simulink model "sgMdl_CAN_J1939Loopback"  (R2024b)
settings: Solver=FixedStepAuto  StartTime=0.0  StopTime=inf  RelTol=1e-3  EnableMultiTasking=on
undefined symbols (not defined in the file): Down, ET1_EMS, IO602, Pull, TCFG2_TECU
libraries: j1939protocollib x8, speedgoatlib_IO602_4 x5, simulink x3, slrtj1939tllib x2
Description:
  | CAN - Working with J1939
settings Model: ModifiedByFormat=Speedgoat  SimulationMode=external  ExtModeEnableFloating=off  ExtModeTrigDuration=100000  VariantFading=off  Creator=Speedgoat  LastModifiedBy=Speedgoat
settings SolverCC: ConcurrentTasks=on  AlgebraicLoopSolver=TrustRegion  PositivePriorityOrder=on  AutoInsertRateTranBlk=on  InsertRTBMode=Never (minimum delay)
settings DataIOCC: SaveFormat=StructureWithTime
settings OptimizationCC: BlockReduction=off  OptimizeBlockIOStorage=off  BufferReuse=off  GlobalBufferReuse=off  ExpressionFolding=off  LocalBlockOutputs=off  OptimizeDataStoreBuffers=off  BusAssignmentInplaceUpdate=off
settings DebuggingCC: InheritedTsInSrcMsg=none  TasksWithSamePriorityMsg=none  ParameterPrecisionLossMsg=none  UnconnectedInputMsg=warning  UnconnectedOutputMsg=warning  UnconnectedLineMsg=warning
settings HardwareCC: ProdBitPerLong=64  ProdLongLongMode=on  ProdHWDeviceType=Intel->x86-64 (Linux 64)
settings ModelReferenceCC: EnableRefExpFcnMdlSchedulingChecks=on
settings SFSimCC: CustomCodeUndefinedFunction=UseInterfaceOnly
settings RTWCC: Description=Speedgoat Real-Time Target Machine  SystemTargetFile=speedgoat.tlc  TemplateMakefile=slrealtime_default_tmf  Toolchain=Simulink Real-Time Toolchain  BuildConfiguration=Faster Runs  TargetLang=C++  GPUComputeCapability=3.5  DLArmComputeVersion=19.05
settings SimulinkRealTimeTargetCC: SubcomponentCodeInterfacePackaging=Reusable function  InstructionSetFMA=off  LogToMDFFile=off  SLRTFileLogMaxRuns=10  UseGCCFastMath=on
settings ConfigComp: CovBoundaryAbsTol=1.0e-5

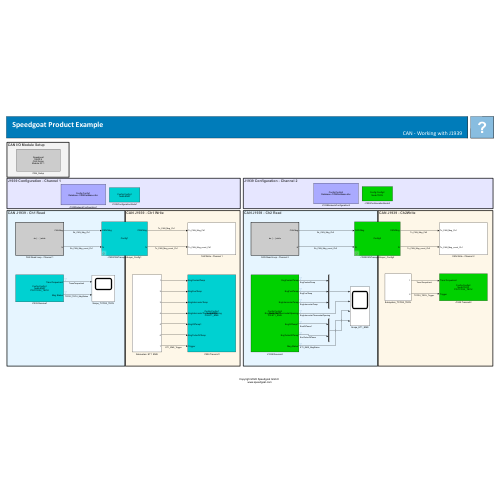
[thumbnail: Simulink's stored preview of the top-level diagram]
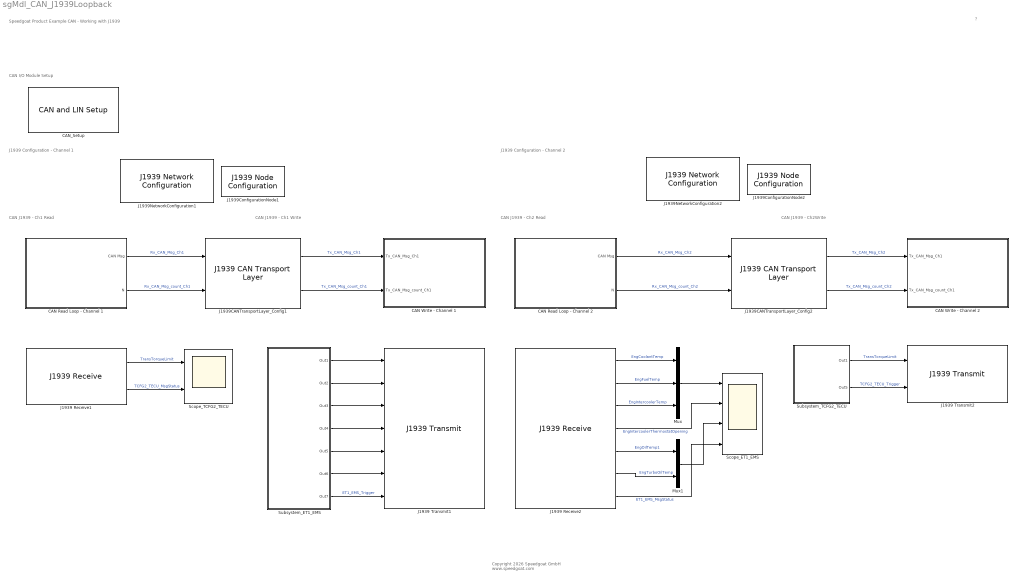
== system sgMdl_CAN_J1939Loopback ==
  note: CAN I/O Module Setup
  note: J1939 Configuration - Channel 1
  note: CAN J1939 - Ch2 Read
  note: CAN J1939 - Ch2Write
  note: CAN J1939 - Ch1 Read
  note: CAN J1939 - Ch1 Write
  note: J1939 Configuration - Channel 2
  note: Speedgoat Product Example
      | CAN - Working with J1939
  note: ?
  note: Copyright 2026 Speedgoat GmbH
      |  www.speedgoat.com
  CAN Read Loop - Channel 1 : Subsystem  TreatAsAtomicUnit=on
  CAN Read Loop - Channel 2 : Subsystem  TreatAsAtomicUnit=on
  CAN Write - Channel 1 : Subsystem
  CAN Write - Channel 2 : Subsystem
  CAN_Setup : speedgoatlib_IO602_4/CAN and LIN Setup   moduleInitValues="[6022     1     1    -1    -1]"  id=1  moduleType=IO602-2  pciSlot=-1  canChn1=CAN (HS)  canChn2=CAN (HS)  canChn3=Disabled  canChn4=Disabled  linChn1=Disabled  linChn2=Disabled  canInitStructArray=[]  canTermStructArray=[]  gpioChnx=Disabled  canChn1InitValues="[2   2   8   1  16   3  19   2   2   5   2   0]"  arbBdrChn1=500 kBaud  clockDividerChn1=Enable  arbManBdrChn1=[8,1,16,3]  fdBdrChn1=5.0 MBaud  fdManBdrChn1=[2,2,5,2]  termResistor1=off  canChn2InitValues="[2   2   8   1  16   3  19   2   2   5   2   0]"  arbBdrChn2=500 kBaud  clockDividerChn2=Enable  arbManBdrChn2=[8,1,16,3]  fdBdrChn2=5.0 MBaud  fdManBdrChn2=[2,2,5,2]  termResistor2=off  canChn3InitValues="[1   0   2   8  31   8  19   2   2   5   2   0]"  arbBdrChn3=1.0 MBaud  clockDividerChn3=Enable  arbManBdrChn3=[2,8,31,8]  fdBdrChn3=5.0 MBaud  fdManBdrChn3=[2,2,5,2]  termResistor3=off  canChn4InitValues="[1   0   2   8  31   8  19   2   2   5   2   0]"  arbBdrChn4=1.0 MBaud  clockDividerChn4=Enable  arbManBdrChn4=[2,8,31,8]  fdBdrChn4=5.0 MBaud  fdManBdrChn4=[2,2,5,2]  termResistor4=off  linChn1InitValues="[0  9600]"  linBtrChn1=9600  linChn2InitValues="[0  9600]"  linBtrChn2=9600  doInitTermStruct="[0  5  0  0  0]"  parDoChannels=[1 2]  parDoVoltage=5  parDoInitValues=0  parDoReset=1  parNumOfDoS=0  parDiChannels=[3 4]  parDiVoltage=5  parDiPull=Pull-Down
      settings: SourceProductName=Simulink Real-Time: Speedgoat I/O Blockset
  J1939 Receive1 : j1939protocollib/J1939 Receive  Priority=-1  ConfigName=Config1  NodeName=EMS  PGList=TCFG2_TECU(65099)  PGName=TCFG2_TECU  MsgLength=8  SignalInfo=TransTorqueLimit$0$16$1$2$1$0$1$0$0$64255$Nm$1845$#  NSignals=1  StartBits=str2num('[double(0)]')  SignalSizes=str2num('[double(16)]')  ByteOrders=str2num('[int32(1)]')  DataTypes=str2num('[int32(2)]')  MultiplexTypes=str2num('[int32(1)]')  MultiplexValues=str2num('[double(0)]')  Factors=str2num('[double(1)]')  Offsets=str2num('[double(0)]')  Minimums=str2num('[double(0)]')  Maximums=str2num('[double(64255)]')  Units=0  SPN=str2num('[double(1845)]')  Comment=0  SrcAddrFilter=Allow all  SrcAddress=255  DestAddrFilter=1  outputNew=on  SampleTime=0.01  ApplyMinMax=off
  J1939 Receive2 : j1939protocollib/J1939 Receive  Priority=-1  ConfigName=Config2  NodeName=TECU  PGList=ET1_EMS(65262)  PGName=ET1_EMS  MsgLength=8  SignalInfo=EngCoolantTemp$0$8$1$2$1$0$1$-40$-40$210$deg$110$#EngFuelTemp$8$8$1$2$1$0$1$-40$-40$210$deg$174$#EngIntercoolerTemp$48$8$1$2$1$0$1$-40$-40$210$deg$52$#EngIntercoolerThermostatOpening$56$8$1$2$1$0$4.000000e-01$0$0$100$%$1134$#EngOilTemp1$16$16$1$2$1$0$3.125000e-02$-273$-273$1735$deg$175$#EngTurboOilTemp$32$16$1$2$1$0$3.125000e-02$-273$-273$1735$deg$176$#  NSignals=6  StartBits=str2num('[double(0);double(8);double(48);double(56);double(16);double(32)]')  SignalSizes=str2num('[double(8),double(8),double(8),double(8),double(16),double(16)]')  ByteOrders=str2num('[int32(1);int32(1);int32(1);int32(1);int32(1);int32(1)]')  DataTypes=str2num('[int32(2);int32(2);int32(2);int32(2);int32(2);int32(2)]')  MultiplexTypes=str2num('[int32(1);int32(1);int32(1);int32(1);int32(1);int32(1)]')  MultiplexValues=str2num('[double(0);double(0);double(0);double(0);double(0);double(0)]')  Factors=str2num('[double(1);double(1);double(1);double(4.000000e-01);double(3.125000e-02);double(3.125000e-02)]')  Offsets=str2num('[double(-40);double(-40);double(-40);double(0);double(-273);double(-273)]')  Minimums=str2num('[double(-40);double(-40);double(-40);double(0);double(-273);double(-273)]')  Maximums=str2num('[double(210);double(210);double(210);double(100);double(1735);double(1735)]')  Units=0  SPN=str2num('[double(110);double(174);double(52);double(1134);double(175);double(176)]')  Comment=0  SrcAddrFilter=Allow all  SrcAddress=255  DestAddrFilter=1  outputNew=on  SampleTime=0.01  ApplyMinMax=off
  J1939 Transmit1 : j1939protocollib/J1939 Transmit  Priority=-1  ConfigName=Config1  NodeName=EMS  PGList=ET1_EMS(65262)  PGName=ET1_EMS  MsgLength=8  SignalInfo=EngCoolantTemp$0$8$1$2$1$0$1$-40$-40$210$deg$110$#EngFuelTemp$8$8$1$2$1$0$1$-40$-40$210$deg$174$#EngIntercoolerTemp$48$8$1$2$1$0$1$-40$-40$210$deg$52$#EngIntercoolerThermostatOpening$56$8$1$2$1$0$4.000000e-01$0$0$100$%$1134$#EngOilTemp1$16$16$1$2$1$0$3.125000e-02$-273$-273$1735$deg$175$#EngTurboOilTemp$32$16$1$2$1$0$3.125000e-02$-273$-273$1735$deg$176$#  NSignals=6  StartBits=str2num('[double(0);double(8);double(48);double(56);double(16);double(32)]')  SignalSizes=str2num('[double(8),double(8),double(8),double(8),double(16),double(16)]')  ByteOrders=str2num('[int32(1);int32(1);int32(1);int32(1);int32(1);int32(1)]')  DataTypes=str2num('[int32(2);int32(2);int32(2);int32(2);int32(2);int32(2)]')  MultiplexTypes=str2num('[int32(1);int32(1);int32(1);int32(1);int32(1);int32(1)]')  MultiplexValues=str2num('[double(0);double(0);double(0);double(0);double(0);double(0)]')  Factors=str2num('[double(1);double(1);double(1);double(4.000000e-01);double(3.125000e-02);double(3.125000e-02)]')  Offsets=str2num('[double(-40);double(-40);double(-40);double(0);double(-273);double(-273)]')  Minimums=str2num('[double(-40);double(-40);double(-40);double(0);double(-273);double(-273)]')  Maximums=str2num('[double(210);double(210);double(210);double(100);double(1735);double(1735)]')  Units=0  SPN=str2num('[double(110);double(174);double(52);double(1134);double(175);double(176)]')  Comment=0  PGPriority=6  DestAddrID=Custom  DestAddrName=255  TransmitPeriodically=on  MessagePeriod=0  SampleTime=-1  ApplyMinMax=off
  J1939 Transmit2 : j1939protocollib/J1939 Transmit  Priority=-1  ConfigName=Config2  NodeName=TECU  PGList=TCFG2_TECU(65099)  PGName=TCFG2_TECU  MsgLength=8  SignalInfo=TransTorqueLimit$0$16$1$2$1$0$1$0$0$64255$Nm$1845$#  NSignals=1  StartBits=str2num('[double(0)]')  SignalSizes=str2num('[double(16)]')  ByteOrders=str2num('[int32(1)]')  DataTypes=str2num('[int32(2)]')  MultiplexTypes=str2num('[int32(1)]')  MultiplexValues=str2num('[double(0)]')  Factors=str2num('[double(1)]')  Offsets=str2num('[double(0)]')  Minimums=str2num('[double(0)]')  Maximums=str2num('[double(64255)]')  Units=0  SPN=str2num('[double(1845)]')  Comment=0  PGPriority=6  DestAddrID=Custom  DestAddrName=255  TransmitPeriodically=on  MessagePeriod=0  SampleTime=-1  ApplyMinMax=off
  J1939CANTransportLayer_Config1 : slrtj1939tllib/J1939 CAN Transport Layer  ConfigNameVal=Config1  SampleTime=-1  MaxCANTx=20
  J1939CANTransportLayer_Config2 : slrtj1939tllib/J1939 CAN Transport Layer  ConfigNameVal=Config2  SampleTime=-1  MaxCANTx=20
  J1939ConfigurationNode1 : j1939protocollib/J1939 Node Configuration  Priority=-2  ConfigName=Config1  NodeID=EMS  NodeName=EMS  PrevNodeID=Custom  PrevConfig=Config  AllowAAC=off  NodeAddress=0  IndustryGroup=0  VehicleSystem=0  VehicleSystemInstance=0  FunctionID=0  FunctionInstance=0  ECUInstance=0  ManufacturerCode=1861  IDNumber=603212  SampleTime=0.01  OutputAddress=off  OutputACStatus=off  enableAC=on
  J1939ConfigurationNode2 : j1939protocollib/J1939 Node Configuration  Priority=-2  ConfigName=Config2  NodeID=TECU  NodeName=TECU  PrevNodeID=Custom  PrevConfig=Config  AllowAAC=off  NodeAddress=3  IndustryGroup=0  VehicleSystem=0  VehicleSystemInstance=0  FunctionID=3  FunctionInstance=0  ECUInstance=0  ManufacturerCode=1861  IDNumber=603214  SampleTime=0.01  OutputAddress=off  OutputACStatus=off  enableAC=on
  J1939NetworkConfiguration1 : j1939protocollib/J1939 Network Configuration  Priority=-3  ConfigName=Config1  DbFile=J1939Database.dbc  PrevDbFile=J1939Database.dbc  enableAC=on
  J1939NetworkConfiguration2 : j1939protocollib/J1939 Network Configuration  Priority=-3  ConfigName=Config2  DbFile=J1939Database.dbc  PrevDbFile=J1939Database.dbc  enableAC=on
  Mux : Mux  Inputs=3
  Mux1 : Mux  Inputs=2
  Scope_ET1_EMS : Scope  NumInputPorts=4
  Scope_TCFG2_TECU : Scope  NumInputPorts=2
  Subsystem_ET1_EMS : Subsystem
  Subsystem_TCFG2_TECU : Subsystem
  wires:
  CAN Read Loop - Channel 2/1(CAN Msg) -> J1939CANTransportLayer_Config2/1  "Rx_CAN_Msg_Ch2"
  CAN Read Loop - Channel 2/2(N) -> J1939CANTransportLayer_Config2/2  "Rx_CAN_Msg_count_Ch2"
  J1939CANTransportLayer_Config2/1 -> CAN Write - Channel 2/1(Tx_CAN_Msg_Ch1)  "Tx_CAN_Msg_Ch2"
  J1939 Receive2/3 -> Mux/3  "EngIntercoolerTemp"
  J1939 Receive2/1 -> Mux/1  "EngCoolantTemp"
  J1939CANTransportLayer_Config2/2 -> CAN Write - Channel 2/2(Tx_CAN_Msg_count_Ch1)  "Tx_CAN_Msg_count_Ch2"
  J1939 Receive2/4 -> Scope_ET1_EMS/2  "EngIntercoolerThermostatOpening"
  J1939 Receive2/2 -> Mux/2  "EngFuelTemp"
  Subsystem_ET1_EMS/4(Out4) -> J1939 Transmit1/4
  Subsystem_ET1_EMS/3(Out3) -> J1939 Transmit1/3
  Subsystem_ET1_EMS/1(Out1) -> J1939 Transmit1/1
  Subsystem_ET1_EMS/2(Out2) -> J1939 Transmit1/2
  CAN Read Loop - Channel 1/2(N) -> J1939CANTransportLayer_Config1/2  "Rx_CAN_Msg_count_Ch1"
  CAN Read Loop - Channel 1/1(CAN Msg) -> J1939CANTransportLayer_Config1/1  "Rx_CAN_Msg_Ch1"
  Subsystem_TCFG2_TECU/1(Out1) -> J1939 Transmit2/1  "TransTorqueLimit"
  Subsystem_TCFG2_TECU/2(Out5) -> J1939 Transmit2/2  "TCFG2_TECU_Trigger"
  J1939 Receive1/1 -> Scope_TCFG2_TECU/1  "TransTorqueLimit"
  Subsystem_ET1_EMS/5(Out5) -> J1939 Transmit1/5
  Subsystem_ET1_EMS/6(Out6) -> J1939 Transmit1/6
  Subsystem_ET1_EMS/7(Out7) -> J1939 Transmit1/7  "ET1_EMS_Trigger"
  J1939 Receive2/5 -> Mux1/1  "EngOilTemp1"
  J1939 Receive2/6 -> Mux1/2  "EngTurboOilTemp"
  Mux/1 -> Scope_ET1_EMS/1
  Mux1/1 -> Scope_ET1_EMS/3
  J1939 Receive2/7 -> Scope_ET1_EMS/4  "ET1_EMS_MsgStatus"
  J1939 Receive1/2 -> Scope_TCFG2_TECU/2  "TCFG2_TECU_MsgStatus"
  J1939CANTransportLayer_Config1/1 -> CAN Write - Channel 1/1(Tx_CAN_Msg_Ch1)  "Tx_CAN_Msg_Ch1"
  J1939CANTransportLayer_Config1/2 -> CAN Write - Channel 1/2(Tx_CAN_Msg_count_Ch1)  "Tx_CAN_Msg_count_Ch1"

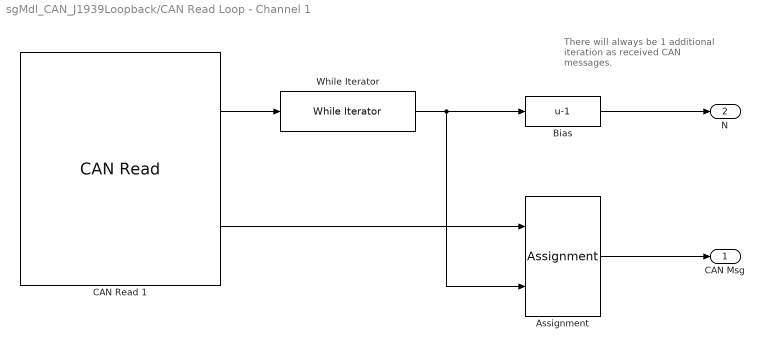
== system sgMdl_CAN_J1939Loopback/CAN Read Loop - Channel 1 ==
  note: There will always be 1 additional iteration as received CAN messages.
  Assignment : Assignment  OutputInitialize=Specify size for each dimension in table  DiagnosticForDimensions=Warning  IndexOptions=Index vector (port)  Indices=1  OutputSizes=501
  Bias : Bias  Bias=-1  SaturateOnIntegerOverflow=off
  CAN Read 1 : speedgoatlib_IO602_4/CAN Read   moduleType=IO602-2  id=1  channel=1  messageType=CAN (HS)  useBusOut=off  HasMulRead=Single Read from Buffer (FIFO)  MsgIDlist=[200,400]  isEFF=off  LabelInHex=off  enableInput=off  initValues=[6022 1 -1 0 1 1 0 0 1 0 2 200 400]  ts=-1
      settings: SourceProductName=Simulink Real-Time: Speedgoat I/O Blockset
  While Iterator : WhileIterator  MaxIters=500  WhileBlockType=do-while  ShowIterationPort=on  OutputDataType=double
  CAN Msg : Outport  VectorParamsAs1DForOutWhenUnconnected=off
  N : Outport  Port=2  VectorParamsAs1DForOutWhenUnconnected=off
  wires:
  CAN Read 1/2 -> Assignment/1
  While Iterator/1 -> Assignment/2, Bias/1
  CAN Read 1/1 -> While Iterator/1
  Assignment/1 -> CAN Msg/1
  Bias/1 -> N/1

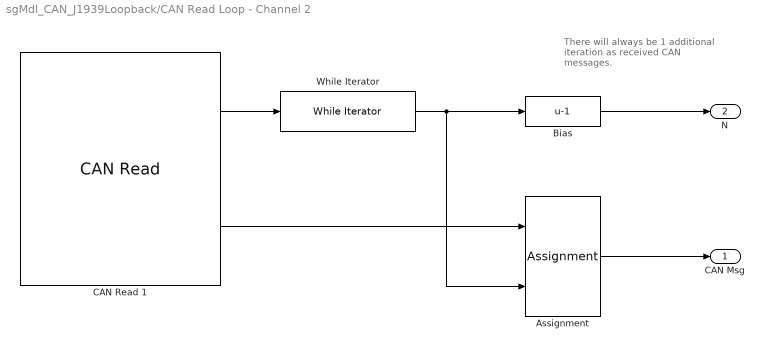
== system sgMdl_CAN_J1939Loopback/CAN Read Loop - Channel 2 ==
  note: There will always be 1 additional iteration as received CAN messages.
  Assignment : Assignment  OutputInitialize=Specify size for each dimension in table  DiagnosticForDimensions=Warning  IndexOptions=Index vector (port)  Indices=1  OutputSizes=501
  Bias : Bias  Bias=-1  SaturateOnIntegerOverflow=off
  CAN Read 1 : speedgoatlib_IO602_4/CAN Read   moduleType=IO602-2  id=1  channel=2  messageType=CAN (HS)  useBusOut=off  HasMulRead=Single Read from Buffer (FIFO)  MsgIDlist=[200,400]  isEFF=off  LabelInHex=off  enableInput=off  initValues=[6022 1 -1 1 1 1 0 0 1 0 2 200 400]  ts=-1
      settings: SourceProductName=Simulink Real-Time: Speedgoat I/O Blockset
  While Iterator : WhileIterator  MaxIters=501  WhileBlockType=do-while  ShowIterationPort=on  OutputDataType=double
  CAN Msg : Outport  VectorParamsAs1DForOutWhenUnconnected=off
  N : Outport  Port=2  VectorParamsAs1DForOutWhenUnconnected=off
  wires:
  Assignment/1 -> CAN Msg/1
  CAN Read 1/1 -> While Iterator/1
  While Iterator/1 -> Bias/1, Assignment/2
  CAN Read 1/2 -> Assignment/1
  Bias/1 -> N/1

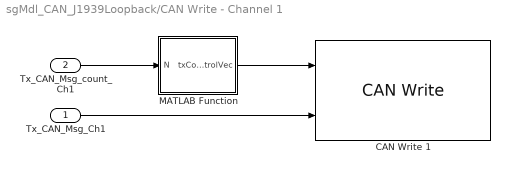
== system sgMdl_CAN_J1939Loopback/CAN Write - Channel 1 ==
  Tx_CAN_Msg_Ch1 : Inport
  Tx_CAN_Msg_count_Ch1 : Inport  Port=2
  CAN Write 1 : speedgoatlib_IO602_4/CAN Write   moduleType=IO602-2  id=1  channel=1  messageType=CAN (HS)  useBusIn=off  numOfMsg=20  enableInput=on  enableStatusPort=off  ts=-1  initValues=[6022 1 -1 0 1 1 0 20 1 0]
      settings: SourceProductName=Simulink Real-Time: Speedgoat I/O Blockset
  MATLAB Function : MATLAB Function  TreatAsAtomicUnit=on  mask(N2TxControlVec){canBusSize=20}
      mask prompts: canBusSize "CAN Bus Size"
      mask help: Speedgoat MATLAB Function Block<br>MATLAB Function - N to Transmission Control Vector<br><br>&copy; 2007 - 2024, Speedgoat GmbH, <a href="matlab: web('www.speedgoat.com','-browser');">www.speedgoat.com</a>
      mask init:
      | sg_mask('MATLAB Function', 'N to Transmission Control Vector', '', 'BlockType', 'MATLAB Function');
  wires:
  MATLAB Function/1(txControlVec) -> CAN Write 1/1
  Tx_CAN_Msg_Ch1/1 -> CAN Write 1/2
  Tx_CAN_Msg_count_Ch1/1 -> MATLAB Function/1(N)

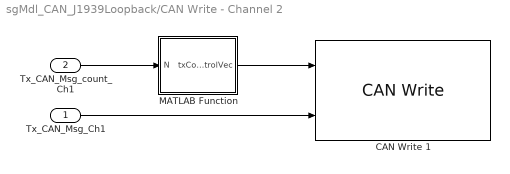
== system sgMdl_CAN_J1939Loopback/CAN Write - Channel 2 ==
  Tx_CAN_Msg_Ch1 : Inport
  Tx_CAN_Msg_count_Ch1 : Inport  Port=2
  CAN Write 1 : speedgoatlib_IO602_4/CAN Write   moduleType=IO602-2  id=1  channel=2  messageType=CAN (HS)  useBusIn=off  numOfMsg=20  enableInput=on  enableStatusPort=off  ts=-1  initValues=[6022 1 -1 1 1 1 0 20 1 0]
      settings: SourceProductName=Simulink Real-Time: Speedgoat I/O Blockset
  MATLAB Function : MATLAB Function  TreatAsAtomicUnit=on  mask(N2TxControlVec){canBusSize=20}
      mask prompts: canBusSize "CAN Bus Size"
      mask help: Speedgoat MATLAB Function Block<br>MATLAB Function - N to Transmission Control Vector<br><br>&copy; 2007 - 2024, Speedgoat GmbH, <a href="matlab: web('www.speedgoat.com','-browser');">www.speedgoat.com</a>
      mask init:
      | sg_mask('MATLAB Function', 'N to Transmission Control Vector', '', 'BlockType', 'MATLAB Function');
  wires:
  MATLAB Function/1(txControlVec) -> CAN Write 1/1
  Tx_CAN_Msg_Ch1/1 -> CAN Write 1/2
  Tx_CAN_Msg_count_Ch1/1 -> MATLAB Function/1(N)

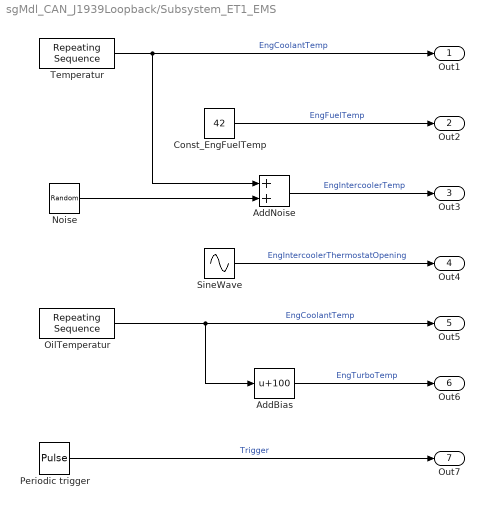
== system sgMdl_CAN_J1939Loopback/Subsystem_ET1_EMS ==
  AddBias : Bias  Bias=100  SaturateOnIntegerOverflow=off
  AddNoise : Sum
  Const_EngFuelTemp : Constant  Value=42  OutDataTypeStr=double  SampleTime=-1
  Noise : RandomNumber  Variance=20
      settings: AttributesFormatString=|
      | Mean: %<Mean>
      | Variance: %<Variance>
  OilTemperatur : simulink/Sources/Repeating Sequence  rep_seq_t=[0 2.5]  rep_seq_y=[-100 1000]
  Periodic trigger : DiscretePulseGenerator  Period=5  SampleTime=0.01
  SineWave : Sin  SineType=Sample based  Amplitude=50  Bias=50  Frequency=2*pi  Samples=250  SampleTime=0.01
  Temperatur : simulink/Sources/Repeating Sequence  rep_seq_t=[0 .5 1 2 2.5]  rep_seq_y=[-40 0 150 210 0]
  Out1 : Outport
  Out2 : Outport  Port=2
  Out3 : Outport  Port=3
  Out4 : Outport  Port=4
  Out5 : Outport  Port=5
  Out6 : Outport  Port=6
  Out7 : Outport  Port=7
  wires:
  AddNoise/1 -> Out3/1  "EngIntercoolerTemp"
  Const_EngFuelTemp/1 -> Out2/1  "EngFuelTemp"
  Temperatur/1 -> AddNoise/1, Out1/1  "EngCoolantTemp"
  SineWave/1 -> Out4/1  "EngIntercoolerThermostatOpening"
  Periodic trigger/1 -> Out7/1  "Trigger"
  Noise/1 -> AddNoise/2
  OilTemperatur/1 -> AddBias/1, Out5/1  "EngCoolantTemp"
  AddBias/1 -> Out6/1  "EngTurboTemp"

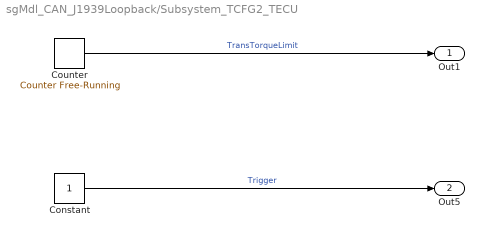
== system sgMdl_CAN_J1939Loopback/Subsystem_TCFG2_TECU ==
  Constant : Constant
  Counter : simulink/Sources/Counter Free-Running  NumBits=16  tsamp=-1
      settings: AttributesFormatString=|
      | ---
      | Limit = %<NumBits> bits
  Out1 : Outport
  Out5 : Outport  Port=2
  wires:
  Constant/1 -> Out5/1  "Trigger"
  Counter/1 -> Out1/1  "TransTorqueLimit"

== matlab function sgMdl_CAN_J1939Loopback/CAN Write - Channel 2/MATLAB Function ==
  data: N input; txControlVec output; canBusSize parameter
function txControlVec = fcn(N, canBusSize)
    txControlVec = zeros(1, canBusSize, 'uint32');
    txControlVec(1:N) = 1;
end

== matlab function sgMdl_CAN_J1939Loopback/CAN Write - Channel 1/MATLAB Function ==
  data: N input; txControlVec output; canBusSize parameter
function txControlVec = fcn(N, canBusSize)
    txControlVec = zeros(1, canBusSize, 'uint32');
    txControlVec(1:N) = 1;
end
